simulink model "Automatic_shifting"  (R2014b)
settings: Solver=ode4  StartTime=0.0  StopTime=inf  RelTol=1e-3
libraries: simulink x4
settings Model: ExtModeTrigDuration=2  Creator=bjoern  LastModifiedBy=bjoern
settings OptimizationCC: OptimizeModelRefInitCode=on  LifeSpan=1
settings DebuggingCC: UnderspecifiedInitializationDetection=Classic  MergeDetectMultiDrivingBlocksExec=none  SolverPrmCheckMsg=none
settings HardwareCC: ProdBitPerInt=16  ProdBitPerPointer=8  ProdIntDivRoundTo=Zero  ProdEndianess=LittleEndian  ProdWordSize=8  ProdHWDeviceType=Atmel->AVR
settings RTWCC: SystemTargetFile=realtime.tlc  GenerateMakefile=off  TemplateMakefile=realtime.tmf  Description=Run on Target Hardware  RTWVerbose=off  ProcessScript=realtime_make_rtw_hook
settings STFCustomTargetCC: TargetLibSuffix=.a  GenerateSampleERTMain=on  ERTCustomFileBanners=on  SupportNonInlinedSFcns=off  SupportVariableSizeSignals=on  MATLABClassNameForMDSCustomization=Simulink.SoftwareTarget.ERTCustomization  GRTInterface=off  SystemTargetFile=realtime.tlc
settings ERTTargetCC: GenerateSampleERTMain=on  ParMdlRefBuildCompliant=off  CompOptLevelCompliant=off  ConcurrentExecutionCompliant=off  CombineOutputUpdateFcns=off  ERTFirstTimeCompliant=off  SupportContinuousTime=on  SupportVariableSizeSignals=on  ModelStepFunctionPrototypeControlCompliant=off  CPPClassGenCompliant=off  ExtModeTransport=3  ExtModeMexFile=ext_serial_win32_comm  ExtModeMexArgs=0 1 9600  InlinedParameterPlacement=NonHierarchical  ERTSrcFileBannerTemplate=realtime_code_template.cgt  ERTHdrFileBannerTemplate=realtime_code_template.cgt  ERTDataSrcFileTemplate=realtime_code_template.cgt  ERTDataHdrFileTemplate=realtime_code_template.cgt  ERTCustomFileTemplate=realtime_file_process.tlc

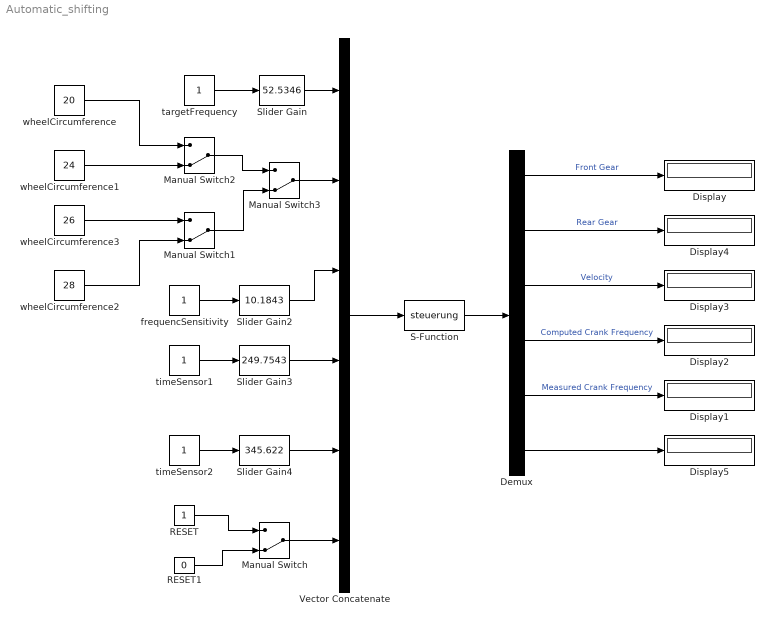
== system Automatic_shifting ==
  Demux : Demux  Outputs=6
  Display{,1..5} (6 alike) : Display
  Manual Switch{,1..3} (4 alike) : ManualSwitch  CurrentSetting=0
  RESET : Constant
  RESET1 : Constant  Value=0
  S-Function : S-Function  FunctionName=steuerung  EnableBusSupport=off
  Slider Gain : simulink/Math Operations/Slider Gain  low=0  gain=52.5346  high=100
  Slider Gain2 : simulink/Math Operations/Slider Gain  low=5  gain=10.1843  high=50
  Slider Gain3 : simulink/Math Operations/Slider Gain  low=90  gain=249.7543  high=2000
  Slider Gain4 : simulink/Math Operations/Slider Gain  low=0  gain=345.622  high=1000
  Vector Concatenate : Concatenate  NumInputs=6
  frequencSensitivity : Constant
  targetFrequency : Constant
  timeSensor1 : Constant
  timeSensor2 : Constant
  wheelCircumference : Constant  Value=20
  wheelCircumference1 : Constant  Value=24
  wheelCircumference2 : Constant  Value=28
  wheelCircumference3 : Constant  Value=26
  wires:
  targetFrequency/1 -> Slider Gain/1
  Vector Concatenate/1 -> S-Function/1
  frequencSensitivity/1 -> Slider Gain2/1
  timeSensor1/1 -> Slider Gain3/1
  timeSensor2/1 -> Slider Gain4/1
  S-Function/1 -> Demux/1
  Demux/3 -> Display3/1  "Velocity"
  Demux/4 -> Display2/1  "Computed Crank Frequency"
  Demux/2 -> Display4/1  "Rear Gear"
  Demux/5 -> Display1/1  "Measured Crank Frequency"
  Demux/1 -> Display/1  "Front Gear"
  Slider Gain/1 -> Vector Concatenate/1
  Slider Gain2/1 -> Vector Concatenate/3
  Slider Gain3/1 -> Vector Concatenate/4
  Slider Gain4/1 -> Vector Concatenate/5
  RESET1/1 -> Manual Switch/2
  RESET/1 -> Manual Switch/1
  Manual Switch/1 -> Vector Concatenate/6
  Demux/6 -> Display5/1
  Manual Switch3/1 -> Vector Concatenate/2
  Manual Switch2/1 -> Manual Switch3/1
  Manual Switch1/1 -> Manual Switch3/2
  wheelCircumference/1 -> Manual Switch2/1
  wheelCircumference1/1 -> Manual Switch2/2
  wheelCircumference2/1 -> Manual Switch1/2
  wheelCircumference3/1 -> Manual Switch1/1
